simulink model "TelemasterTrimLin"  (R2024b)
settings: Solver=ode4  StartTime=0.0  StopTime=t(end)  FixedStep=dt  RelTol=1e-3
libraries: Telemaster_Lib x1
settings Model: Creator=igmso  LastModifiedBy=MASTER
settings DataIOCC: ExternalInput=[t,u]  InitialState=getstatestruct(SteadyState(cont).op)  LoadExternalInput=on  LoadInitialState=on  SaveFormat=StructureWithTime
settings RTWCC: GPUComputeCapability=3.5

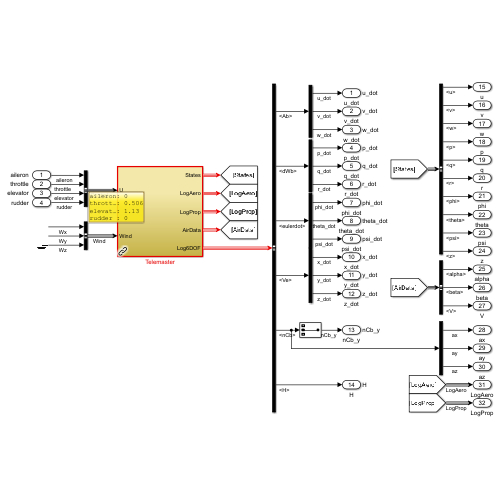
[thumbnail: Simulink's stored preview of the top-level diagram]
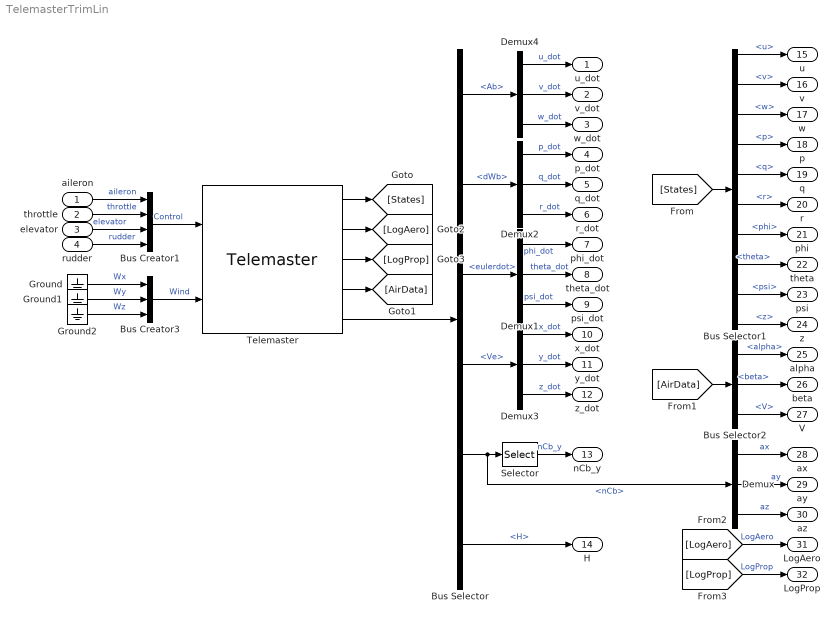
== system TelemasterTrimLin ==
  aileron : Inport  Unit=deg
  throttle : Inport  Port=2  Unit=%
  elevator : Inport  Port=3  Unit=deg
  rudder : Inport  Port=4  Unit=deg
  Bus Creator3 : BusCreator  Inputs=3
  Bus Selector : BusSelector  OutputSignals=Ab,dWb,eulerdot,Ve,nCb,H
  Bus Selector1 : BusSelector  OutputSignals=u,v,w,p,q,r,phi,theta,psi,z
  Bus Selector2 : BusSelector  OutputSignals=alpha,beta,V
  Bus Creator1 : BusCreator  Inputs=4
  Demux{,1..4} (5 alike) : Demux  Outputs=3
  Ground : Ground
  Ground1 : Ground
  Ground2 : Ground
  Selector : Selector  InputPortWidth=3  IndexOptions=Index vector (dialog)  Indices=2  OutputSizes=1
  Telemaster : Telemaster_Lib/Telemaster  SystemSampleTime=-1  VariantActivationTime=update diagram  AllowFlexibleInterface=on  Latency=0  AutoFrameSizeCalculation=off
  u_dot : Outport  SignalName=u_dot  Unit=m/s^2
  v_dot : Outport  Port=2  SignalName=v_dot  Unit=m/s^2
  w_dot : Outport  Port=3  SignalName=w_dot  Unit=m/s^2
  p_dot : Outport  Port=4  SignalName=p_dot
  q_dot : Outport  Port=5  SignalName=q_dot
  r_dot : Outport  Port=6  SignalName=r_dot
  phi_dot : Outport  Port=7  SignalName=phi_dot
  theta_dot : Outport  Port=8  SignalName=theta_dot
  psi_dot : Outport  Port=9  SignalName=psi_dot
  x_dot : Outport  Port=10  SignalName=x_dot
  y_dot : Outport  Port=11  SignalName=y_dot
  z_dot : Outport  Port=12  SignalName=z_dot
  nCb_y : Outport  Port=13  SignalName=nCb_y
  H : Outport  Port=14  SignalName=H
  u : Outport  Port=15
  v : Outport  Port=16
  w : Outport  Port=17
  p : Outport  Port=18
  q : Outport  Port=19
  r : Outport  Port=20
  phi : Outport  Port=21
  theta : Outport  Port=22
  psi : Outport  Port=23
  z : Outport  Port=24
  alpha : Outport  Port=25
  beta : Outport  Port=26
  V : Outport  Port=27
  ax : Outport  Port=28
  ay : Outport  Port=29
  az : Outport  Port=30
  LogAero : Outport  Port=31
  LogProp : Outport  Port=32
  wires:
  Ground/1 -> Bus Creator3/1  "Wx"
  Ground1/1 -> Bus Creator3/2  "Wy"
  Ground2/1 -> Bus Creator3/3  "Wz"
  Bus Creator1/1 -> Telemaster/1  "Control"
  Bus Creator3/1 -> Telemaster/2  "Wind"
  Telemaster/1 -> [States]
  Telemaster/5 -> Bus Selector/1
  Bus Selector/1 -> Demux4/1  "<Ab>"
  Bus Selector/2 -> Demux2/1  "<dWb>"
  Bus Selector/3 -> Demux1/1  "<eulerdot>"
  Bus Selector/4 -> Demux3/1  "<Ve>"
  Demux1/1 -> phi_dot/1  "phi_dot"
  Demux1/3 -> psi_dot/1  "psi_dot"
  Demux3/2 -> y_dot/1  "y_dot"
  Demux1/2 -> theta_dot/1  "theta_dot"
  Demux3/1 -> x_dot/1  "x_dot"
  Demux3/3 -> z_dot/1  "z_dot"
  Telemaster/4 -> [AirData]
  Demux2/1 -> p_dot/1  "p_dot"
  Demux2/2 -> q_dot/1  "q_dot"
  Demux2/3 -> r_dot/1  "r_dot"
  Demux4/1 -> u_dot/1  "u_dot"
  Demux4/2 -> v_dot/1  "v_dot"
  Demux4/3 -> w_dot/1  "w_dot"
  Bus Selector/5 -> Demux/1, Selector/1  "<nCb>"
  Selector/1 -> nCb_y/1  "nCb_y"
  Bus Selector/6 -> H/1  "<H>"
  aileron/1 -> Bus Creator1/1  "aileron"
  throttle/1 -> Bus Creator1/2  "throttle"
  rudder/1 -> Bus Creator1/4  "rudder"
  Telemaster/2 -> [LogAero]
  Telemaster/3 -> [LogProp]
  [States] -> Bus Selector1/1
  Bus Selector1/9 -> psi/1  "<psi>"
  Bus Selector1/10 -> z/1  "<z>"
  Bus Selector1/7 -> phi/1  "<phi>"
  Bus Selector1/8 -> theta/1  "<theta>"
  Bus Selector1/6 -> r/1  "<r>"
  Bus Selector1/4 -> p/1  "<p>"
  Bus Selector1/3 -> w/1  "<w>"
  Bus Selector1/1 -> u/1  "<u>"
  Bus Selector1/5 -> q/1  "<q>"
  Bus Selector1/2 -> v/1  "<v>"
  [AirData] -> Bus Selector2/1
  Bus Selector2/3 -> V/1  "<V>"
  Bus Selector2/2 -> beta/1  "<beta>"
  Bus Selector2/1 -> alpha/1  "<alpha>"
  Demux/3 -> az/1  "az"
  Demux/2 -> ay/1  "ay"
  Demux/1 -> ax/1  "ax"
  elevator/1 -> Bus Creator1/3  "elevator"
  [LogProp] -> LogProp/1  "LogProp"
  [LogAero] -> LogAero/1  "LogAero"
